simulink model "bal_main___"  (R2015a)
settings: Solver=ode45  StartTime=0.0  StopTime=250  RelTol=1e-3
values from neighbouring files (symbols this model uses):
  Alfa_zad = [-2. 0. 2. 4.5]    [Object_2.m]
  Cxa_pol = [0.042163159  0.060088192  0.082569042  0.11957579 ... (first row only)    [Object_2.m]
  Cya_pol = [0.55431394  0.67438192  0.77265832  0.88446777 ... (first row only)    [Object_2.m]
  h_zad = [0.10 0.15 0.20 0.40 0.60 1.00 3.]    [Object_2.m]
  mz_Alfa = [0.57380685    0.67948784    0.76621719     0.87587322 ... (first row only)    [Object_2.m]
  xt_zad = [0. 0.2326 0.4653 0.698 0.9313 1.164 1.3966 1.6293]    [Object_2.m]
undefined symbols (not defined in the file or in its folder): Cxa_Delta_1, Cxa_Delta_2, Cxa_Delta_3, Cya_Delta_1, Cya_Delta_2, Cya_Delta_3, Delta_1_zad, Delta_2_zad, Delta_3_zad, h_zad_D1_D2, h_zad_D3, mz_Delta_1, mz_Delta_2, mz_Delta_3
libraries: simulink x6
settings Model: Creator=Admin  LastModifiedBy=Гена

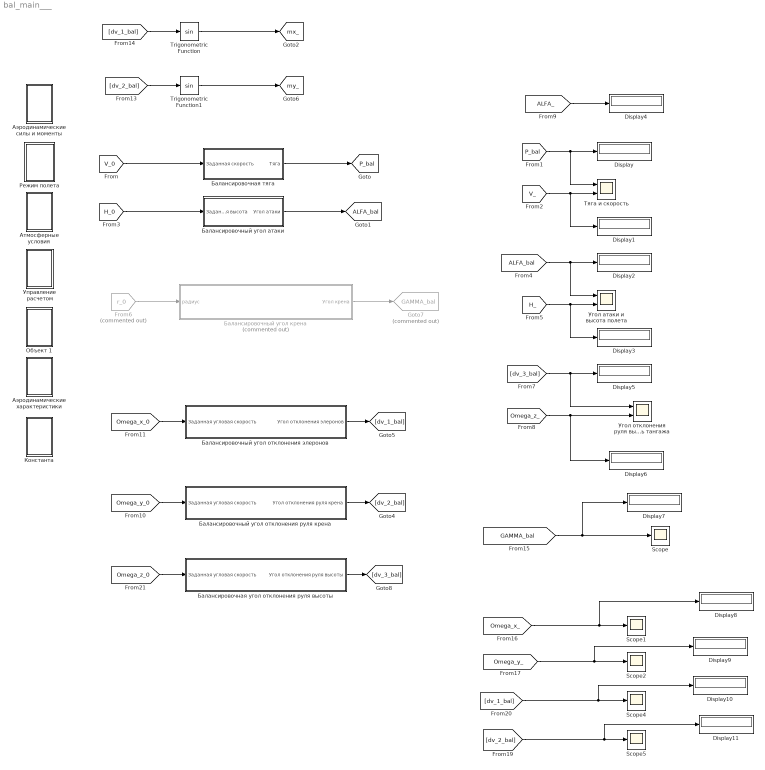
== system bal_main___ ==
  Display{,1..11} (12 alike) : Display
  From6 : From  Commented=on  GotoTag=r_0  TagVisibility=global
  Goto7 : Goto  Commented=on  GotoTag=GAMMA_bal  TagVisibility=global
  Scope{,1..2,4..5} (5 alike) : Scope
      Scope settings: YMin=4999.71  YMax=4999.79  SaveName=ScopeData6
      Scope1 settings: YMin=-7700  YMax=-6700  SaveName=ScopeData7
      Scope2 settings: YMin=-7.5  YMax=7.5  SaveName=ScopeData8
      Scope4 settings: YMin=-29000  YMax=-27900  SaveName=ScopeData9
      Scope5 settings: SaveName=ScopeData10
  Trigonometric Function : Trigonometry
  Trigonometric Function1 : Trigonometry
  Атмосферные условия : Subsystem
  Аэродинамические характеристики : Subsystem
  Аэродинамические силы и моменты : Subsystem
  Балансировочная угол отклонения руля высоты : Subsystem
  Балансировочная тяга : Subsystem
  Балансировочный угол атаки : Subsystem
  Балансировочный угол крена : Subsystem  Commented=on
  Балансировочный угол отклонения руля крена : Subsystem
  "Балансировочный угол отклонения элеронов " : Subsystem
  Константа : Subsystem
  Объект 1 : Subsystem
  Режим полета : Subsystem  mask(Параметры исходного полета){M_LA=1000, V_0=100, H_0=0.5, r_0=0.5, omega_x=0, omega_y=0, omega_z=0, Psi_0=0}
      mask prompts: M_LA "Полетная масса, кг"; V_0 "Скорость полета, м/с"; H_0 "Высота полета, м"; r_0 "Радиус разворота, м"; omega_x "Угловая скорость x"; omega_y "Угловая скорость y"; omega_z "Угловая скорость z"; Psi_0 "Угол пси"
  "Тяга и скорость " : Scope  NumInputPorts=2
      settings: TimeRange=100  YMin=0~20  YMax=7000~55
  Угол атаки и высота полета : Scope  NumInputPorts=2
      settings: TimeRange=100  YMin=-5.208~0.49991  YMax=-5.195~0.50009
  Угол отклонения руля высоты и угловая скорость тангажа : Scope  NumInputPorts=2
      settings: TimeRange=100  YMin=-6~-5  YMax=14~5  SaveName=ScopeData2
  Управление расчетом : Subsystem
  tag scope: ALFA_bal=global, P_bal=global, mx_=global, my_=global
  wires:
  [V_0] -> Балансировочная тяга/1(Заданная скорость)
  Балансировочная тяга/1(Тяга) -> [P_bal]
  [P_bal] -> Display/1, "Тяга и скорость "/1
  [V_] -> Display1/1, "Тяга и скорость "/2
  [H_0] -> Балансировочный угол атаки/1(Заданная высота)
  Балансировочный угол атаки/1(Угол атаки) -> [ALFA_bal]
  [ALFA_bal] -> Display2/1, Угол атаки и высота полета/1
  [H_] -> Display3/1, Угол атаки и высота полета/2
  [dv_3_bal] -> Display5/1, Угол отклонения руля высоты и угловая скорость тангажа/1
  [Omega_z_] -> Display6/1, Угол отклонения руля высоты и угловая скорость тангажа/2
  [ALFA_] -> Display4/1
  [dv_2_bal] -> Trigonometric Function1/1
  [dv_1_bal] -> Trigonometric Function/1
  [Omega_y_0] -> Балансировочный угол отклонения руля крена/1(Заданная угловая скорость)
  [Omega_x_0] -> "Балансировочный угол отклонения элеронов "/1(Заданная угловая скорость)
  Балансировочный угол отклонения руля крена/1(Угол отклонения руля крена) -> [dv_2_bal]
  "Балансировочный угол отклонения элеронов "/1(Угол отклонения элеронов) -> [dv_1_bal]
  [Omega_y_] -> Display9/1, Scope2/1
  [Omega_x_] -> Display8/1, Scope1/1
  [GAMMA_bal] -> Display7/1, Scope/1
  [dv_1_bal] -> Display10/1, Scope4/1
  [Omega_z_0] -> Балансировочная угол отклонения руля высоты/1(Заданная угловая скорость)
  Балансировочная угол отклонения руля высоты/1(Угол отклонения руля высоты) -> [dv_3_bal]
  Trigonometric Function/1 -> [mx_]
  Trigonometric Function1/1 -> [my_]
  From6/1 -> Балансировочный угол крена/1(радиус)
  [dv_2_bal] -> Display11/1, Scope5/1
  Балансировочный угол крена/1("Угол крена ") -> Goto7/1

== system bal_main___/Атмосферные условия ==
  Плотность : Constant  Value=1.225
  tag scope: Ro=global
  wires:
  Плотность/1 -> [Ro]

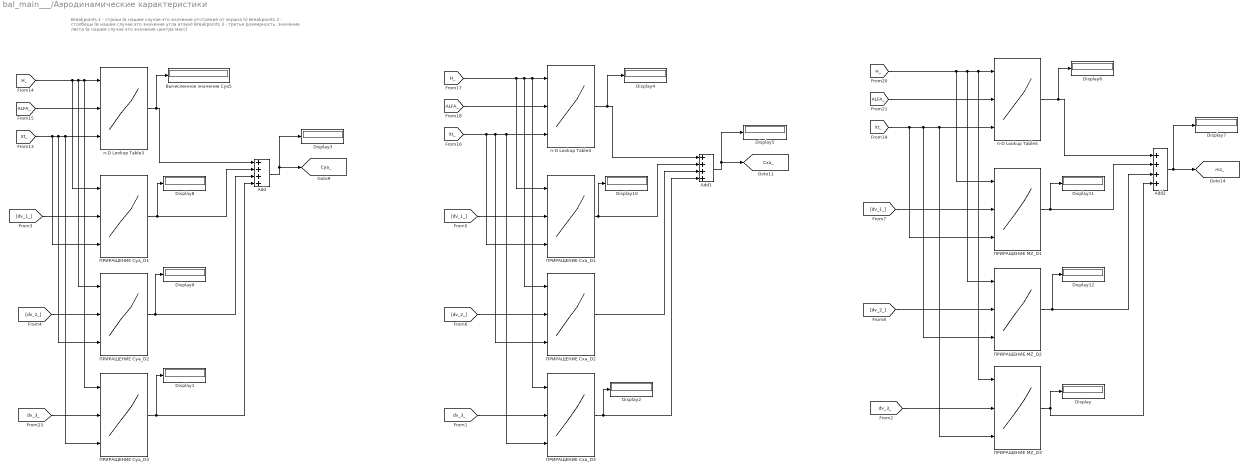
== system bal_main___/Аэродинамические характеристики ==
  note: Breakpoints 1 - строки (в нашем случае это значение отстояния от экрана h)
      | Breakpoints 2 - столбецы (в нашем случае это значение угла атаки)
      | Breakpoints 3 - третья размерность, значение листа (в нашем случае это значение центра масс)
  Add : Sum  Inputs=++++
  Add1 : Sum  Inputs=++++
  Add2 : Sum  Inputs=++++
  Display{,1..12} (13 alike) : Display
  n-D Lookup Table3 : Lookup_n-D  NumberOfTableDimensions=3  BreakpointsForDimension1=h_zad  BreakpointsForDimension2=Alfa_zad  BreakpointsForDimension3=xt_zad  Table=Cya_pol  InternalRulePriority=Speed  RndMeth=Simplest  InputSameDT=on
  n-D Lookup Table4 : Lookup_n-D  NumberOfTableDimensions=3  BreakpointsForDimension1=h_zad  BreakpointsForDimension2=Alfa_zad  BreakpointsForDimension3=xt_zad  Table=Cxa_pol  InternalRulePriority=Speed  RndMeth=Simplest  InputSameDT=on
  n-D Lookup Table5 : Lookup_n-D  NumberOfTableDimensions=3  BreakpointsForDimension1=h_zad  BreakpointsForDimension2=Alfa_zad  BreakpointsForDimension3=xt_zad  Table=mz_Alfa  InternalRulePriority=Speed  RndMeth=Simplest  InputSameDT=on
  Вычисленное значение Суа5 : Display
  ПРИРАЩЕНИЕ Cxa_D1 : Lookup_n-D  NumberOfTableDimensions=3  BreakpointsForDimension1=h_zad_D1_D2  BreakpointsForDimension2=Delta_1_zad  BreakpointsForDimension3=xt_zad  Table=Cxa_Delta_1  InternalRulePriority=Speed  RndMeth=Simplest  InputSameDT=on
  ПРИРАЩЕНИЕ Cxa_D2 : Lookup_n-D  NumberOfTableDimensions=3  BreakpointsForDimension1=h_zad_D1_D2  BreakpointsForDimension2=Delta_2_zad  BreakpointsForDimension3=xt_zad  Table=Cxa_Delta_2  InternalRulePriority=Speed  RndMeth=Simplest  InputSameDT=on
  ПРИРАЩЕНИЕ Cxa_D3 : Lookup_n-D  NumberOfTableDimensions=3  BreakpointsForDimension1=h_zad_D3  BreakpointsForDimension2=Delta_3_zad  BreakpointsForDimension3=xt_zad  Table=Cxa_Delta_3  InternalRulePriority=Speed  RndMeth=Simplest  InputSameDT=on
  ПРИРАЩЕНИЕ Cya_D1 : Lookup_n-D  NumberOfTableDimensions=3  BreakpointsForDimension1=h_zad_D1_D2  BreakpointsForDimension2=Delta_1_zad  BreakpointsForDimension3=xt_zad  Table=Cya_Delta_1  InternalRulePriority=Speed  RndMeth=Simplest  InputSameDT=on
  ПРИРАЩЕНИЕ Cya_D2 : Lookup_n-D  NumberOfTableDimensions=3  BreakpointsForDimension1=h_zad_D1_D2  BreakpointsForDimension2=Delta_2_zad  BreakpointsForDimension3=xt_zad  Table=Cya_Delta_2  InternalRulePriority=Speed  RndMeth=Simplest  InputSameDT=on
  ПРИРАЩЕНИЕ Cya_D3 : Lookup_n-D  NumberOfTableDimensions=3  BreakpointsForDimension1=h_zad_D3  BreakpointsForDimension2=Delta_3_zad  BreakpointsForDimension3=xt_zad  Table=Cya_Delta_3  InternalRulePriority=Speed  RndMeth=Simplest  InputSameDT=on
  ПРИРАЩЕНИЕ MZ_D1 : Lookup_n-D  NumberOfTableDimensions=3  BreakpointsForDimension1=h_zad_D1_D2  BreakpointsForDimension2=Delta_1_zad  BreakpointsForDimension3=xt_zad  Table=mz_Delta_1  InternalRulePriority=Speed  RndMeth=Simplest  InputSameDT=on
  ПРИРАЩЕНИЕ MZ_D2 : Lookup_n-D  NumberOfTableDimensions=3  BreakpointsForDimension1=h_zad_D1_D2  BreakpointsForDimension2=Delta_2_zad  BreakpointsForDimension3=xt_zad  Table=mz_Delta_2  InternalRulePriority=Speed  RndMeth=Simplest  InputSameDT=on
  ПРИРАЩЕНИЕ MZ_D3 : Lookup_n-D  NumberOfTableDimensions=3  BreakpointsForDimension1=h_zad_D3  BreakpointsForDimension2=Delta_3_zad  BreakpointsForDimension3=xt_zad  Table=mz_Delta_3  InternalRulePriority=Speed  RndMeth=Simplest  InputSameDT=on
  tag scope: Cxa_=global, Cya_=global, mz_=global
  wires:
  [H_] -> ПРИРАЩЕНИЕ Cya_D3/1, n-D Lookup Table3/1, ПРИРАЩЕНИЕ Cya_D2/1, ПРИРАЩЕНИЕ Cya_D1/1
  [Xt_] -> ПРИРАЩЕНИЕ Cya_D2/3, ПРИРАЩЕНИЕ Cya_D3/3, n-D Lookup Table3/3, ПРИРАЩЕНИЕ Cya_D1/3
  n-D Lookup Table3/1 -> Вычисленное значение Суа5/1, Add/1
  [H_] -> ПРИРАЩЕНИЕ Cxa_D1/1, ПРИРАЩЕНИЕ Cxa_D2/1, ПРИРАЩЕНИЕ Cxa_D3/1, n-D Lookup Table4/1
  [Xt_] -> ПРИРАЩЕНИЕ Cxa_D1/3, ПРИРАЩЕНИЕ Cxa_D2/3, n-D Lookup Table4/3, ПРИРАЩЕНИЕ Cxa_D3/3
  [ALFA_] -> n-D Lookup Table5/2
  [ALFA_] -> n-D Lookup Table4/2
  [ALFA_] -> n-D Lookup Table3/2
  [Xt_] -> ПРИРАЩЕНИЕ MZ_D1/3, ПРИРАЩЕНИЕ MZ_D2/3, n-D Lookup Table5/3, ПРИРАЩЕНИЕ MZ_D3/3
  [dv_3_] -> ПРИРАЩЕНИЕ Cxa_D3/2
  Add/1 -> Display3/1, [Cya_]
  n-D Lookup Table4/1 -> Display4/1, Add1/1
  Add1/1 -> Display5/1, [Cxa_]
  n-D Lookup Table5/1 -> Display6/1, Add2/1
  Add2/1 -> Display7/1, [mz_]
  [dv_3_] -> ПРИРАЩЕНИЕ MZ_D3/2
  [dv_1_] -> ПРИРАЩЕНИЕ Cya_D1/2
  [dv_2_] -> ПРИРАЩЕНИЕ Cya_D2/2
  ПРИРАЩЕНИЕ Cya_D1/1 -> Display8/1, Add/2
  ПРИРАЩЕНИЕ Cya_D2/1 -> Display9/1, Add/3
  [dv_3_] -> ПРИРАЩЕНИЕ Cya_D3/2
  ПРИРАЩЕНИЕ Cya_D3/1 -> Display1/1, Add/4
  ПРИРАЩЕНИЕ Cxa_D3/1 -> Display2/1, Add1/4
  [dv_1_] -> ПРИРАЩЕНИЕ Cxa_D1/2
  ПРИРАЩЕНИЕ Cxa_D1/1 -> Display10/1, Add1/2
  [dv_2_] -> ПРИРАЩЕНИЕ Cxa_D2/2
  ПРИРАЩЕНИЕ Cxa_D2/1 -> Add1/3
  ПРИРАЩЕНИЕ MZ_D3/1 -> Add2/4, Display/1
  [dv_1_] -> ПРИРАЩЕНИЕ MZ_D1/2
  ПРИРАЩЕНИЕ MZ_D1/1 -> Display11/1, Add2/2
  [H_] -> ПРИРАЩЕНИЕ MZ_D2/1, ПРИРАЩЕНИЕ MZ_D3/1, n-D Lookup Table5/1, ПРИРАЩЕНИЕ MZ_D1/1
  [dv_2_] -> ПРИРАЩЕНИЕ MZ_D2/2
  ПРИРАЩЕНИЕ MZ_D2/1 -> Display12/1, Add2/3

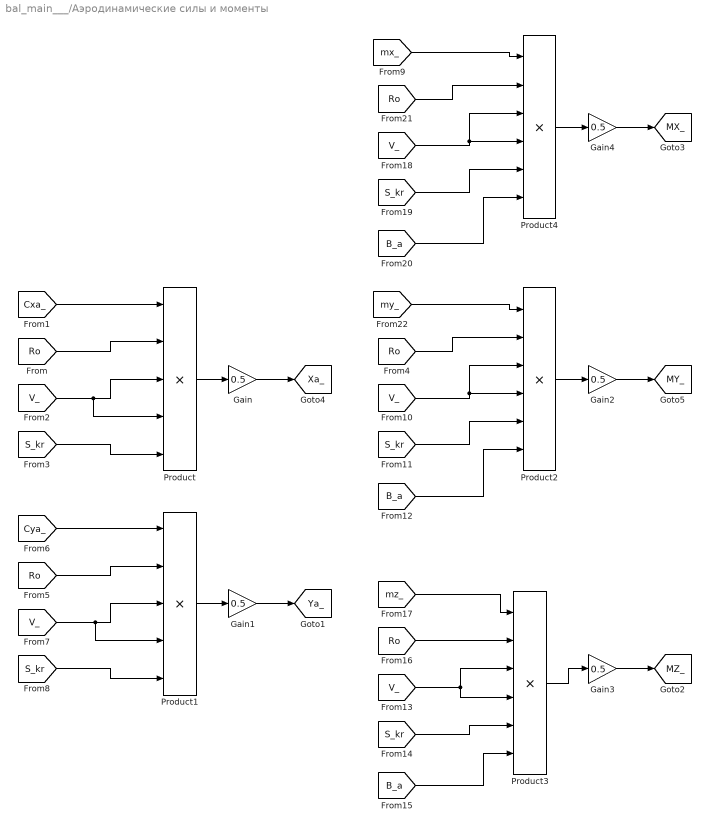
== system bal_main___/Аэродинамические силы и моменты ==
  Gain{,1..4} (5 alike) : Gain  Gain=0.5
  Product : Product  Inputs=*****
  Product1 : Product  Inputs=*****
  Product2 : Product  Inputs=******
  Product3 : Product  Inputs=******
  Product4 : Product  Inputs=******
  tag scope: MX_=global, MY_=global, MZ_=global, Xa_=global, Ya_=global
  wires:
  Product/1 -> Gain/1
  [S_kr] -> Product/5
  Gain/1 -> [Xa_]
  [Cxa_] -> Product/1
  [Ro] -> Product/2
  [V_] -> Product/4, Product/3
  Product1/1 -> Gain1/1
  [S_kr] -> Product1/5
  Gain1/1 -> [Ya_]
  [Cya_] -> Product1/1
  [Ro] -> Product1/2
  [V_] -> Product1/4, Product1/3
  Product2/1 -> Gain2/1
  [S_kr] -> Product2/5
  Gain2/1 -> [MY_]
  [my_] -> Product2/1
  [Ro] -> Product2/2
  [B_a] -> Product2/6
  [V_] -> Product2/4, Product2/3
  Product3/1 -> Gain3/1
  [S_kr] -> Product3/5
  Gain3/1 -> [MZ_]
  [mz_] -> Product3/1
  [Ro] -> Product3/2
  [B_a] -> Product3/6
  [V_] -> Product3/4, Product3/3
  Product4/1 -> Gain4/1
  [S_kr] -> Product4/5
  Gain4/1 -> [MX_]
  [mx_] -> Product4/1
  [Ro] -> Product4/2
  [B_a] -> Product4/6
  [V_] -> Product4/4, Product4/3

== system bal_main___/Балансировочная угол отклонения руля высоты ==
  Заданная угловая скорость : Inport
  Add : Sum  Inputs=+-
  Gain : Gain  Gain=-1
  PID Controller : simulink/Continuous/PID Controller  Controller=PID  TimeDomain=Continuous-time  SampleTime=-1  IntegratorMethod=Forward Euler  FilterMethod=Forward Euler  Form=Parallel  UseFilter=on  ControllerParametersSource=internal  P=0.379810440708384  I=0.0731035476397683  D=-0.0897634019475152  N=1.4222540202283  InitialConditionSource=internal  InitialConditionForIntegrator=0  InitialConditionForFilter=0  ExternalReset=none  LimitOutput=off  UpperSaturationLimit=inf  LowerSaturationLimit=-inf  LinearizeAsGain=on  AntiWindupMode=none  Kb=1  TrackingMode=off  Kt=1  PParamMin=[]  PParamMax=[]  IParamMin=[]  IParamMax=[]  DParamMin=[]  DParamMax=[]  NParamMin=[]  NParamMax=[]  KbParamMin=[]  KbParamMax=[]  KtParamMin=[]  KtParamMax=[]  POutMin=[]  POutMax=[]  IOutMin=[]  IOutMax=[]  DOutMin=[]  DOutMax=[]  NOutMin=[]  NOutMax=[]  KbOutMin=[]  KbOutMax=[]  KtOutMin=[]  KtOutMax=[]  IntegratorOutMin=[]  IntegratorOutMax=[]  FilterOutMin=[]  FilterOutMax=[]  SumOutMin=[]  SumOutMax=[]  SumI1OutMin=[]  SumI1OutMax=[]  SumI2OutMin=[]  SumI2OutMax=[]  SumI3OutMin=[]  SumI3OutMax=[]  SumDOutMin=[]  SumDOutMax=[]  SaturationOutMin=[]  SaturationOutMax=[]  IntegratorContinuousStateAttributes=''  IntegratorStateMustResolveToSignalObject=off  IntegratorRTWStateStorageClass=Auto  FilterContinuousStateAttributes=''  FilterStateMustResolveToSignalObject=off  FilterRTWStateStorageClass=Auto  DifferentiatorICPrevScaledInput=0  DifferentiatorOutMin=[]  DifferentiatorOutMax=[]
  Управление угловой скоростью тангажа : Subsystem
  Угол отклонения руля высоты : Outport
  tag scope: Omega_z_=global
  wires:
  Add/1 -> PID Controller/1
  Заданная угловая скорость/1 -> Add/1
  Управление угловой скоростью тангажа/1(Угловая скорость тангажа) -> Add/2, [Omega_z_]
  PID Controller/1 -> Gain/1
  Gain/1 -> Угол отклонения руля высоты/1, Управление угловой скоростью тангажа/1(Угол отклонения руля высоты)

== system bal_main___/Балансировочная тяга ==
  Заданная скорость : Inport
  Add : Sum  Inputs=+-
  PID Controller : simulink/Continuous/PID Controller  Controller=PID  TimeDomain=Continuous-time  SampleTime=-1  IntegratorMethod=Forward Euler  FilterMethod=Forward Euler  Form=Parallel  UseFilter=on  ControllerParametersSource=internal  P=200  I=10  D=1  N=10  InitialConditionSource=internal  InitialConditionForIntegrator=0  InitialConditionForFilter=0  ExternalReset=none  LimitOutput=off  UpperSaturationLimit=inf  LowerSaturationLimit=-inf  LinearizeAsGain=on  AntiWindupMode=none  Kb=1  TrackingMode=off  Kt=1  PParamMin=[]  PParamMax=[]  IParamMin=[]  IParamMax=[]  DParamMin=[]  DParamMax=[]  NParamMin=[]  NParamMax=[]  KbParamMin=[]  KbParamMax=[]  KtParamMin=[]  KtParamMax=[]  POutMin=[]  POutMax=[]  IOutMin=[]  IOutMax=[]  DOutMin=[]  DOutMax=[]  NOutMin=[]  NOutMax=[]  KbOutMin=[]  KbOutMax=[]  KtOutMin=[]  KtOutMax=[]  IntegratorOutMin=[]  IntegratorOutMax=[]  FilterOutMin=[]  FilterOutMax=[]  SumOutMin=[]  SumOutMax=[]  SumI1OutMin=[]  SumI1OutMax=[]  SumI2OutMin=[]  SumI2OutMax=[]  SumI3OutMin=[]  SumI3OutMax=[]  SumDOutMin=[]  SumDOutMax=[]  SaturationOutMin=[]  SaturationOutMax=[]  IntegratorContinuousStateAttributes=''  IntegratorStateMustResolveToSignalObject=off  IntegratorRTWStateStorageClass=Auto  FilterContinuousStateAttributes=''  FilterStateMustResolveToSignalObject=off  FilterRTWStateStorageClass=Auto  DifferentiatorICPrevScaledInput=0  DifferentiatorOutMin=[]  DifferentiatorOutMax=[]
  Управление скоростью : Subsystem
  Тяга : Outport
  tag scope: V_=global
  wires:
  PID Controller/1 -> Тяга/1, Управление скоростью/1(Тяга)
  Add/1 -> PID Controller/1
  Заданная скорость/1 -> Add/1
  Управление скоростью/1(Скорость) -> Add/2, [V_]

== system bal_main___/Балансировочный угол атаки ==
  Заданная высота : Inport
  Add : Sum  Inputs=+-
  PID Controller : simulink/Continuous/PID Controller  Controller=PID  TimeDomain=Continuous-time  SampleTime=-1  IntegratorMethod=Forward Euler  FilterMethod=Forward Euler  Form=Parallel  UseFilter=on  ControllerParametersSource=internal  P=10  I=10  D=10  N=10  InitialConditionSource=internal  InitialConditionForIntegrator=0  InitialConditionForFilter=0  ExternalReset=none  LimitOutput=off  UpperSaturationLimit=inf  LowerSaturationLimit=-inf  LinearizeAsGain=on  AntiWindupMode=none  Kb=1  TrackingMode=off  Kt=1  PParamMin=[]  PParamMax=[]  IParamMin=[]  IParamMax=[]  DParamMin=[]  DParamMax=[]  NParamMin=[]  NParamMax=[]  KbParamMin=[]  KbParamMax=[]  KtParamMin=[]  KtParamMax=[]  POutMin=[]  POutMax=[]  IOutMin=[]  IOutMax=[]  DOutMin=[]  DOutMax=[]  NOutMin=[]  NOutMax=[]  KbOutMin=[]  KbOutMax=[]  KtOutMin=[]  KtOutMax=[]  IntegratorOutMin=[]  IntegratorOutMax=[]  FilterOutMin=[]  FilterOutMax=[]  SumOutMin=[]  SumOutMax=[]  SumI1OutMin=[]  SumI1OutMax=[]  SumI2OutMin=[]  SumI2OutMax=[]  SumI3OutMin=[]  SumI3OutMax=[]  SumDOutMin=[]  SumDOutMax=[]  SaturationOutMin=[]  SaturationOutMax=[]  IntegratorContinuousStateAttributes=''  IntegratorStateMustResolveToSignalObject=off  IntegratorRTWStateStorageClass=Auto  FilterContinuousStateAttributes=''  FilterStateMustResolveToSignalObject=off  FilterRTWStateStorageClass=Auto  DifferentiatorICPrevScaledInput=0  DifferentiatorOutMin=[]  DifferentiatorOutMax=[]
  Управление высотой : Subsystem
  Угол атаки : Outport
  tag scope: H_=global
  wires:
  PID Controller/1 -> Управление высотой/1(Угол атаки), Угол атаки/1
  Add/1 -> PID Controller/1
  Заданная высота/1 -> Add/1
  Управление высотой/1(Высота) -> Add/2, [H_]

== system bal_main___/Балансировочный угол крена ==
  радиус : Inport
  Add1 : Sum  Inputs=+-
  PID Controller : simulink/Continuous/PID Controller  Controller=PID  TimeDomain=Continuous-time  SampleTime=-1  IntegratorMethod=Forward Euler  FilterMethod=Forward Euler  Form=Parallel  UseFilter=on  ControllerParametersSource=internal  P=10  I=0  D=0  N=10  InitialConditionSource=internal  InitialConditionForIntegrator=0  InitialConditionForFilter=0  ExternalReset=none  LimitOutput=off  UpperSaturationLimit=inf  LowerSaturationLimit=-inf  LinearizeAsGain=on  AntiWindupMode=none  Kb=1  TrackingMode=off  Kt=1  PParamMin=[]  PParamMax=[]  IParamMin=[]  IParamMax=[]  DParamMin=[]  DParamMax=[]  NParamMin=[]  NParamMax=[]  KbParamMin=[]  KbParamMax=[]  KtParamMin=[]  KtParamMax=[]  POutMin=[]  POutMax=[]  IOutMin=[]  IOutMax=[]  DOutMin=[]  DOutMax=[]  NOutMin=[]  NOutMax=[]  KbOutMin=[]  KbOutMax=[]  KtOutMin=[]  KtOutMax=[]  IntegratorOutMin=[]  IntegratorOutMax=[]  FilterOutMin=[]  FilterOutMax=[]  SumOutMin=[]  SumOutMax=[]  SumI1OutMin=[]  SumI1OutMax=[]  SumI2OutMin=[]  SumI2OutMax=[]  SumI3OutMin=[]  SumI3OutMax=[]  SumDOutMin=[]  SumDOutMax=[]  SaturationOutMin=[]  SaturationOutMax=[]  IntegratorContinuousStateAttributes=''  IntegratorStateMustResolveToSignalObject=off  IntegratorRTWStateStorageClass=Auto  FilterContinuousStateAttributes=''  FilterStateMustResolveToSignalObject=off  FilterRTWStateStorageClass=Auto  DifferentiatorICPrevScaledInput=0  DifferentiatorOutMin=[]  DifferentiatorOutMax=[]
  Scope : Scope
      settings: SaveName=ScopeData11
  Управление радиусом поворота : Subsystem
  "Угол крена " : Outport
  tag scope: R_=global
  wires:
  радиус/1 -> Add1/1
  PID Controller/1 -> "Угол крена "/1, Управление радиусом поворота/1(Угол крена), Scope/1
  Add1/1 -> PID Controller/1
  Управление радиусом поворота/1(Радиус) -> Add1/2, [R_]

== system bal_main___/Балансировочный угол отклонения руля крена ==
  Заданная угловая скорость : Inport
  Add : Sum  Inputs=+-
  Gain : Gain  Gain=-1
  PID Controller : simulink/Continuous/PID Controller  Controller=PID  TimeDomain=Continuous-time  SampleTime=-1  IntegratorMethod=Forward Euler  FilterMethod=Forward Euler  Form=Parallel  UseFilter=on  ControllerParametersSource=internal  P=0.379810440708384  I=0.0731035476397683  D=-0.0897634019475152  N=1.4222540202283  InitialConditionSource=internal  InitialConditionForIntegrator=0  InitialConditionForFilter=0  ExternalReset=none  LimitOutput=off  UpperSaturationLimit=inf  LowerSaturationLimit=-inf  LinearizeAsGain=on  AntiWindupMode=none  Kb=1  TrackingMode=off  Kt=1  PParamMin=[]  PParamMax=[]  IParamMin=[]  IParamMax=[]  DParamMin=[]  DParamMax=[]  NParamMin=[]  NParamMax=[]  KbParamMin=[]  KbParamMax=[]  KtParamMin=[]  KtParamMax=[]  POutMin=[]  POutMax=[]  IOutMin=[]  IOutMax=[]  DOutMin=[]  DOutMax=[]  NOutMin=[]  NOutMax=[]  KbOutMin=[]  KbOutMax=[]  KtOutMin=[]  KtOutMax=[]  IntegratorOutMin=[]  IntegratorOutMax=[]  FilterOutMin=[]  FilterOutMax=[]  SumOutMin=[]  SumOutMax=[]  SumI1OutMin=[]  SumI1OutMax=[]  SumI2OutMin=[]  SumI2OutMax=[]  SumI3OutMin=[]  SumI3OutMax=[]  SumDOutMin=[]  SumDOutMax=[]  SaturationOutMin=[]  SaturationOutMax=[]  IntegratorContinuousStateAttributes=''  IntegratorStateMustResolveToSignalObject=off  IntegratorRTWStateStorageClass=Auto  FilterContinuousStateAttributes=''  FilterStateMustResolveToSignalObject=off  FilterRTWStateStorageClass=Auto  DifferentiatorICPrevScaledInput=0  DifferentiatorOutMin=[]  DifferentiatorOutMax=[]
  Управление угловой скоростью рыскания : Subsystem
  Угол отклонения руля крена : Outport
  tag scope: Omega_y_=global
  wires:
  Add/1 -> PID Controller/1
  Заданная угловая скорость/1 -> Add/1
  Управление угловой скоростью рыскания/1(Угловая скорость тангажа) -> Add/2, [Omega_y_]
  PID Controller/1 -> Gain/1
  Gain/1 -> Угол отклонения руля крена/1, Управление угловой скоростью рыскания/1(Угол отклонения руля направления)

== system bal_main___/Балансировочный угол отклонения элеронов  ==
  Заданная угловая скорость : Inport
  Add : Sum  Inputs=+-
  Gain : Gain  Gain=-1
  PID Controller : simulink/Continuous/PID Controller  Controller=PID  TimeDomain=Continuous-time  SampleTime=-1  IntegratorMethod=Forward Euler  FilterMethod=Forward Euler  Form=Parallel  UseFilter=on  ControllerParametersSource=internal  P=0.379810440708384  I=0.0731035476397683  D=-0.0897634019475152  N=1.4222540202283  InitialConditionSource=internal  InitialConditionForIntegrator=0  InitialConditionForFilter=0  ExternalReset=none  LimitOutput=off  UpperSaturationLimit=inf  LowerSaturationLimit=-inf  LinearizeAsGain=on  AntiWindupMode=none  Kb=1  TrackingMode=off  Kt=1  PParamMin=[]  PParamMax=[]  IParamMin=[]  IParamMax=[]  DParamMin=[]  DParamMax=[]  NParamMin=[]  NParamMax=[]  KbParamMin=[]  KbParamMax=[]  KtParamMin=[]  KtParamMax=[]  POutMin=[]  POutMax=[]  IOutMin=[]  IOutMax=[]  DOutMin=[]  DOutMax=[]  NOutMin=[]  NOutMax=[]  KbOutMin=[]  KbOutMax=[]  KtOutMin=[]  KtOutMax=[]  IntegratorOutMin=[]  IntegratorOutMax=[]  FilterOutMin=[]  FilterOutMax=[]  SumOutMin=[]  SumOutMax=[]  SumI1OutMin=[]  SumI1OutMax=[]  SumI2OutMin=[]  SumI2OutMax=[]  SumI3OutMin=[]  SumI3OutMax=[]  SumDOutMin=[]  SumDOutMax=[]  SaturationOutMin=[]  SaturationOutMax=[]  IntegratorContinuousStateAttributes=''  IntegratorStateMustResolveToSignalObject=off  IntegratorRTWStateStorageClass=Auto  FilterContinuousStateAttributes=''  FilterStateMustResolveToSignalObject=off  FilterRTWStateStorageClass=Auto  DifferentiatorICPrevScaledInput=0  DifferentiatorOutMin=[]  DifferentiatorOutMax=[]
  Управление угловой скоростью тангажа : Subsystem
  Угол отклонения элеронов : Outport
  tag scope: Omega_x_=global
  wires:
  Add/1 -> PID Controller/1
  Заданная угловая скорость/1 -> Add/1
  Управление угловой скоростью тангажа/1(Угловая скорость крена) -> Add/2, [Omega_x_]
  PID Controller/1 -> Gain/1
  Gain/1 -> Угол отклонения элеронов/1, Управление угловой скоростью тангажа/1(Угол отклонения элеронов)

== system bal_main___/Константа ==
  RAD : Constant  Value=57.3
  g : Constant  Value=9.81
  tag scope: RAD=global, g_=global
  wires:
  g/1 -> [g_]
  RAD/1 -> [RAD]

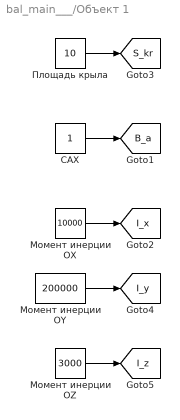
== system bal_main___/Объект 1 ==
  Момент инерции ОX : Constant  Value=10000
  Момент инерции ОY : Constant  Value=200000
  Момент инерции ОZ : Constant  Value=3000
  Площадь крыла : Constant  Value=10
  САХ : Constant
  tag scope: B_a=global, I_x=global, I_y=global, I_z=global, S_kr=global
  wires:
  Площадь крыла/1 -> [S_kr]
  САХ/1 -> [B_a]
  Момент инерции ОX/1 -> [I_x]
  Момент инерции ОY/1 -> [I_y]
  Момент инерции ОZ/1 -> [I_z]

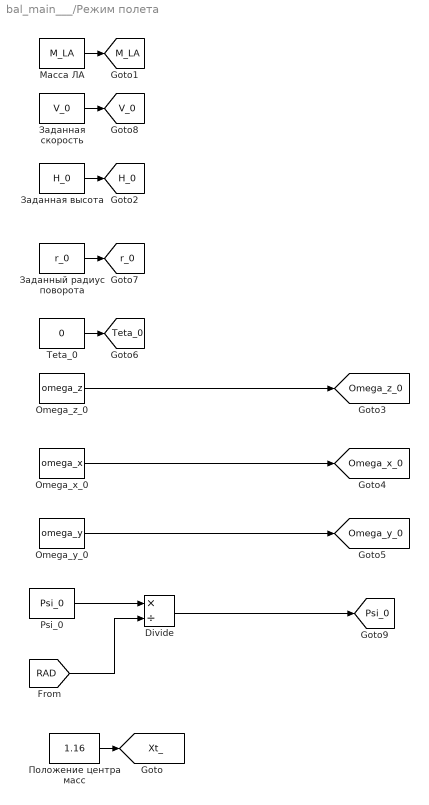
== system bal_main___/Режим полета ==
  Divide : Product  Inputs=*/
  Omega_x_0 : Constant  Value=omega_x
  Omega_y_0 : Constant  Value=omega_y
  Omega_z_0 : Constant  Value=omega_z
  Psi_0 : Constant  Value=Psi_0
  Teta_0 : Constant  Value=0
  Заданная высота : Constant  Value=H_0
  Заданная скорость : Constant  Value=V_0
  Заданный радиус поворота : Constant  Value=r_0
  Масса ЛА : Constant  Value=M_LA
  Положение центра масс : Constant  Value=1.16
  tag scope: H_0=global, M_LA=global, Omega_x_0=global, Omega_y_0=global, Omega_z_0=global, Psi_0=global, Teta_0=global, V_0=global, Xt_=global, r_0=global
  wires:
  Заданная скорость/1 -> [V_0]
  Teta_0/1 -> [Teta_0]
  Масса ЛА/1 -> [M_LA]
  Заданная высота/1 -> [H_0]
  Omega_z_0/1 -> [Omega_z_0]
  Положение центра масс/1 -> [Xt_]
  Omega_x_0/1 -> [Omega_x_0]
  Omega_y_0/1 -> [Omega_y_0]
  Заданный радиус поворота/1 -> [r_0]
  Psi_0/1 -> Divide/1
  Divide/1 -> [Psi_0]
  [RAD] -> Divide/2

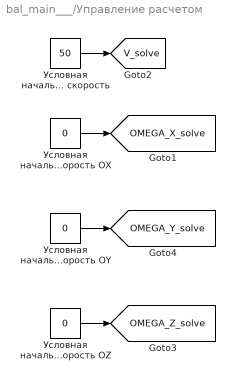
== system bal_main___/Управление расчетом ==
  Условная начальная скорость : Constant  Value=50
  Условная начальная угловая скорость OX : Constant  Value=0
  Условная начальная угловая скорость OY : Constant  Value=0
  Условная начальная угловая скорость OZ : Constant  Value=0
  tag scope: OMEGA_X_solve=global, OMEGA_Y_solve=global, OMEGA_Z_solve=global, V_solve=global
  wires:
  Условная начальная скорость/1 -> [V_solve]
  Условная начальная угловая скорость OX/1 -> [OMEGA_X_solve]
  Условная начальная угловая скорость OZ/1 -> [OMEGA_Z_solve]
  Условная начальная угловая скорость OY/1 -> [OMEGA_Y_solve]

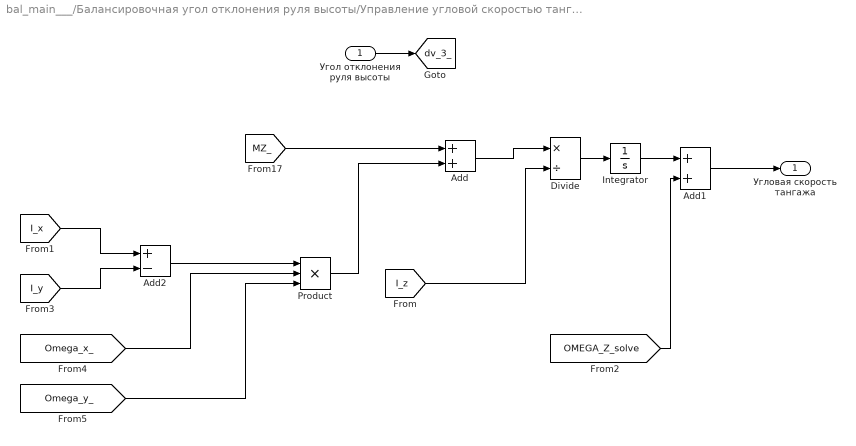
== system bal_main___/Балансировочная угол отклонения руля высоты/Управление угловой скоростью тангажа ==
  Угол отклонения руля высоты : Inport
  Add : Sum
  Add1 : Sum
  Add2 : Sum  Inputs=+-
  Divide : Product  Inputs=*/
  Integrator : Integrator
  Product : Product  Inputs=3
  Угловая скорость тангажа : Outport
  tag scope: dv_3_=global
  wires:
  Угол отклонения руля высоты/1 -> [dv_3_]
  [I_z] -> Divide/2
  Divide/1 -> Integrator/1
  Integrator/1 -> Add1/1
  [OMEGA_Z_solve] -> Add1/2
  Add1/1 -> Угловая скорость тангажа/1
  [MZ_] -> Add/1
  Add/1 -> Divide/1
  [I_x] -> Add2/1
  [I_y] -> Add2/2
  Add2/1 -> Product/1
  Product/1 -> Add/2
  [Omega_x_] -> Product/2
  [Omega_y_] -> Product/3

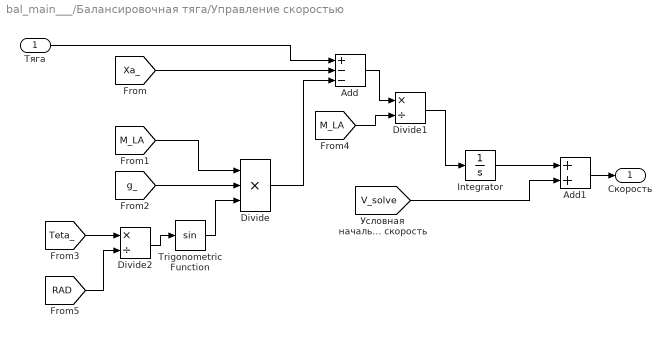
== system bal_main___/Балансировочная тяга/Управление скоростью ==
  Тяга : Inport
  Add : Sum  Inputs=+--
  Add1 : Sum
  Divide : Product  Inputs=***
  Divide1 : Product  Inputs=*/
  Divide2 : Product  Inputs=*/
  Integrator : Integrator
  Trigonometric Function : Trigonometry
  Скорость : Outport
  wires:
  [Xa_] -> Add/2
  Тяга/1 -> Add/1
  [M_LA] -> Divide1/2
  Divide/1 -> Add/3
  Divide1/1 -> Integrator/1
  [M_LA] -> Divide/1
  Trigonometric Function/1 -> Divide/3
  [g_] -> Divide/2
  Add/1 -> Divide1/1
  Add1/1 -> Скорость/1
  Integrator/1 -> Add1/1
  [V_solve] -> Add1/2
  [Teta_] -> Divide2/1
  Divide2/1 -> Trigonometric Function/1
  [RAD] -> Divide2/2

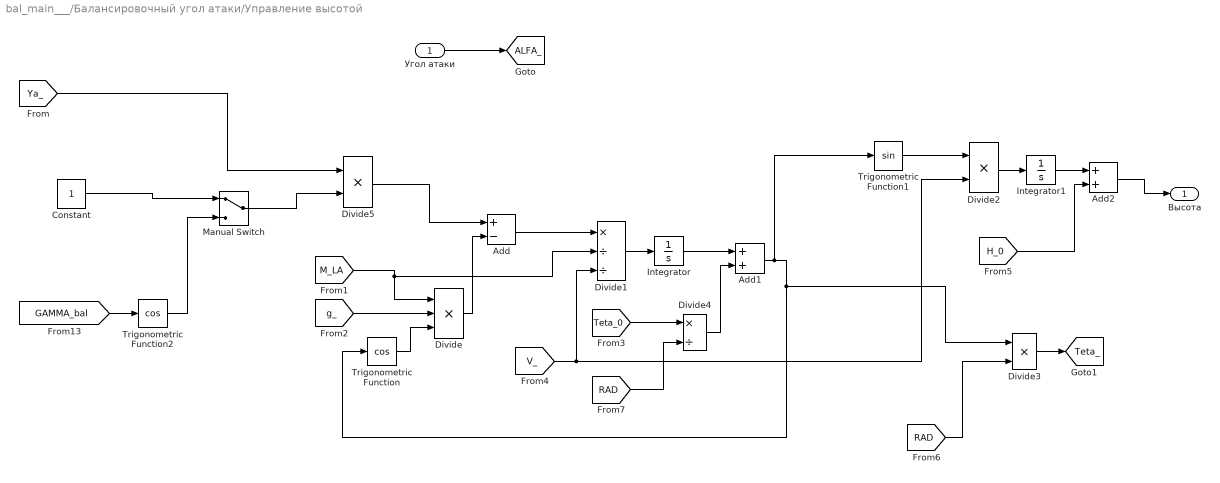
== system bal_main___/Балансировочный угол атаки/Управление высотой ==
  Угол атаки : Inport
  Add : Sum  Inputs=+-
  Add1 : Sum
  Add2 : Sum
  Constant : Constant
  Divide : Product  Inputs=***
  Divide1 : Product  Inputs=*//
  Divide2 : Product  Inputs=**
  Divide3 : Product  Inputs=**
  Divide4 : Product  Inputs=*/
  Divide5 : Product  Inputs=**
  Integrator : Integrator
  Integrator1 : Integrator
  Manual Switch : ManualSwitch
  Trigonometric Function : Trigonometry  Operator=cos
  Trigonometric Function1 : Trigonometry
  Trigonometric Function2 : Trigonometry  Operator=cos
  Высота : Outport
  tag scope: ALFA_=global, Teta_=global
  wires:
  [M_LA] -> Divide1/2, Divide/1
  Trigonometric Function/1 -> Divide/3
  [g_] -> Divide/2
  Divide/1 -> Add/2
  Add/1 -> Divide1/1
  [V_] -> Divide2/2, Divide1/3
  Divide1/1 -> Integrator/1
  Integrator/1 -> Add1/1
  Add1/1 -> Trigonometric Function/1, Divide3/1, Trigonometric Function1/1
  Trigonometric Function1/1 -> Divide2/1
  Divide2/1 -> Integrator1/1
  Integrator1/1 -> Add2/1
  [H_0] -> Add2/2
  Add2/1 -> Высота/1
  Угол атаки/1 -> [ALFA_]
  Divide3/1 -> [Teta_]
  [RAD] -> Divide3/2
  [Teta_0] -> Divide4/1
  Divide4/1 -> Add1/2
  [RAD] -> Divide4/2
  [GAMMA_bal] -> Trigonometric Function2/1
  [Ya_] -> Divide5/1
  Divide5/1 -> Add/1
  Manual Switch/1 -> Divide5/2
  Trigonometric Function2/1 -> Manual Switch/2
  Constant/1 -> Manual Switch/1

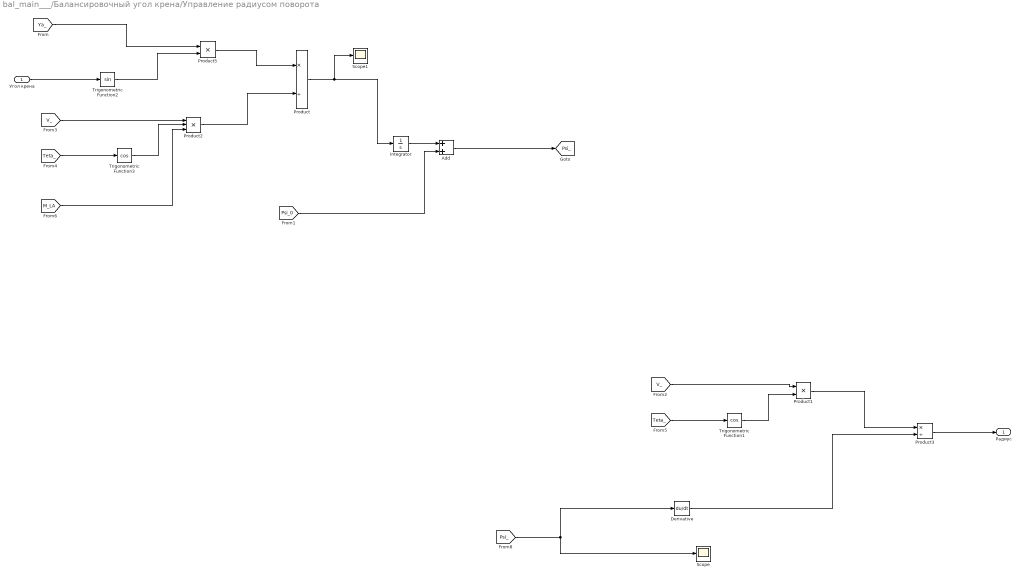
== system bal_main___/Балансировочный угол крена/Управление радиусом поворота ==
  Угол крена : Inport
  Add : Sum
  Derivative : Derivative
  Integrator : Integrator
  Product : Product  Inputs=*/
  Product1 : Product
  Product2 : Product  Inputs=3
  Product3 : Product  Inputs=*/
  Product5 : Product
  Scope : Scope
      settings: SaveName=ScopeData4
  Scope1 : Scope
      settings: SaveName=ScopeData5
  Trigonometric Function1 : Trigonometry  Operator=cos
  Trigonometric Function2 : Trigonometry
  Trigonometric Function3 : Trigonometry  Operator=cos
  Радиус : Outport
  tag scope: Psi_=global
  wires:
  Integrator/1 -> Add/1
  [Psi_0] -> Add/2
  Add/1 -> [Psi_]
  Trigonometric Function3/1 -> Product2/2
  [V_] -> Product2/1
  [Teta_] -> Trigonometric Function3/1
  Product2/1 -> Product/2
  [M_LA] -> Product2/3
  Product/1 -> Integrator/1, Scope1/1
  [Psi_] -> Derivative/1, Scope/1
  Product5/1 -> Product/1
  Trigonometric Function2/1 -> Product5/2
  [Ya_] -> Product5/1
  Угол крена/1 -> Trigonometric Function2/1
  Trigonometric Function1/1 -> Product1/2
  [V_] -> Product1/1
  [Teta_] -> Trigonometric Function1/1
  Product1/1 -> Product3/1
  Derivative/1 -> Product3/2
  Product3/1 -> Радиус/1

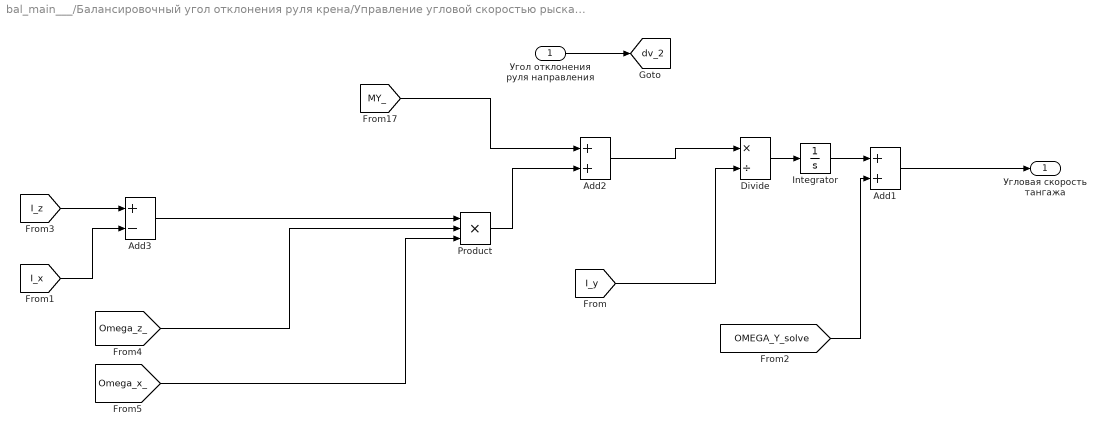
== system bal_main___/Балансировочный угол отклонения руля крена/Управление угловой скоростью рыскания ==
  Угол отклонения руля направления : Inport
  Add1 : Sum
  Add2 : Sum
  Add3 : Sum  Inputs=+-
  Divide : Product  Inputs=*/
  Integrator : Integrator
  Product : Product  Inputs=3
  Угловая скорость тангажа : Outport
  tag scope: dv_2=global
  wires:
  Угол отклонения руля направления/1 -> [dv_2]
  [I_y] -> Divide/2
  Divide/1 -> Integrator/1
  Integrator/1 -> Add1/1
  [OMEGA_Y_solve] -> Add1/2
  Add1/1 -> Угловая скорость тангажа/1
  [MY_] -> Add2/1
  Product/1 -> Add2/2
  Add2/1 -> Divide/1
  [I_z] -> Add3/1
  [I_x] -> Add3/2
  Add3/1 -> Product/1
  [Omega_z_] -> Product/2
  [Omega_x_] -> Product/3

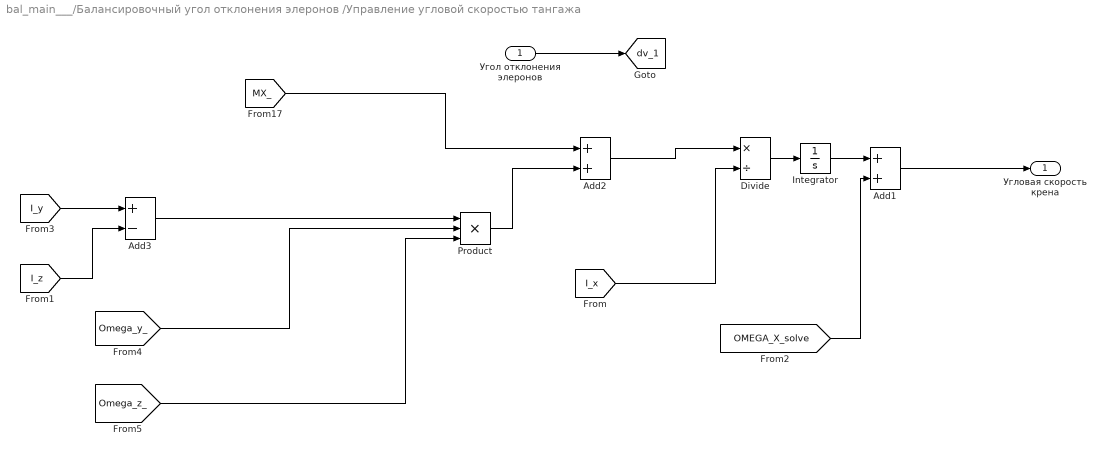
== system bal_main___/Балансировочный угол отклонения элеронов /Управление угловой скоростью тангажа ==
  Угол отклонения элеронов : Inport
  Add1 : Sum
  Add2 : Sum
  Add3 : Sum  Inputs=+-
  Divide : Product  Inputs=*/
  Integrator : Integrator
  Product : Product  Inputs=3
  Угловая скорость крена : Outport
  tag scope: dv_1=global
  wires:
  Угол отклонения элеронов/1 -> [dv_1]
  [I_x] -> Divide/2
  Divide/1 -> Integrator/1
  Integrator/1 -> Add1/1
  [OMEGA_X_solve] -> Add1/2
  Add1/1 -> Угловая скорость крена/1
  [MX_] -> Add2/1
  Product/1 -> Add2/2
  Add2/1 -> Divide/1
  [I_y] -> Add3/1
  [I_z] -> Add3/2
  Add3/1 -> Product/1
  [Omega_y_] -> Product/2
  [Omega_z_] -> Product/3
